simulink model "lab5"  (R2017b)
settings: Solver=VariableStepAuto  StartTime=0.0  StopTime=10  RelTol=1e-3
undefined symbols (not defined in the file or in its folder): c, k, m
settings Model: Creator=ayushi  LastModifiedBy=ayushi

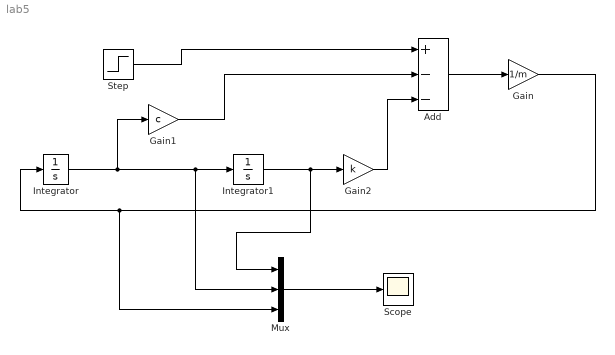
== system lab5 ==
  Add : Sum  Inputs=+--
  Gain : Gain  Gain=1/m
  Gain1 : Gain  Gain=c
  Gain2 : Gain  Gain=k
  Integrator : Integrator
  Integrator1 : Integrator
  Mux : Mux  Inputs=3
  Scope : Scope
  Step : Step  SampleTime=0
  wires:
  Step/1 -> Add/1
  Gain/1 -> Mux/3, Integrator/1
  Add/1 -> Gain/1
  Gain1/1 -> Add/2
  Gain2/1 -> Add/3
  Mux/1 -> Scope/1
  Integrator1/1 -> Mux/1, Gain2/1
  Integrator/1 -> Mux/2, Integrator1/1, Gain1/1
